simulink model "buffer_tut1"  (Simulink 5.0)
settings: Solver=FixedStepDiscrete  StartTime=0.0  StopTime=10.0  RelTol=1e-3
libraries: dspbuff3 x1, dspxfrm3 x1, dspsrcs4 x1
settings Model: CovMetricSettings=d  Creator=ckamachi  LastModifiedBy=ckamachi  ExtModeTrigMode=oneshot  ExtModeArmWhenConnect=off  LimitDataPoints=off  BlockReductionOpt=off  BooleanDataType=off

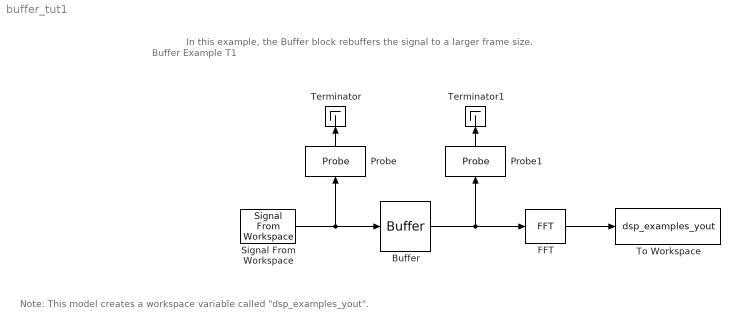
== system buffer_tut1 ==
  note: Buffer Example T1
  note: In this example, the Buffer block rebuffers the signal to a larger frame size.
  note: Note: This model creates a workspace variable called "dsp_examples_yout".
  Buffer : dspbuff3/Buffer  N=16  V=0  ic=0
  FFT : dspxfrm3/FFT  CompMethod=Table lookup  TableOpt=Speed  BitRevOrder=off
  Probe : Probe  Orientation=up  ProbeWidth=off  ProbeComplexSignal=off
  Probe1 : Probe  Orientation=up  ProbeWidth=off  ProbeComplexSignal=off
  Signal From Workspace : dspsrcs4/Signal From Workspace  X=1:1000  Ts=0.125  nsamps=8  OutputAfterFinalValue=Setting to zero
  Terminator : Terminator
      settings: Orientation=up
  Terminator1 : Terminator
      settings: Orientation=up
  To Workspace : ToWorkspace  VariableName=dsp_examples_yout  SampleTime=-1  SaveFormat=Array
  wires:
  FFT/1 -> To Workspace/1
  Signal From Workspace/1 -> Buffer/1, Probe/1
  Buffer/1 -> FFT/1, Probe1/1
  Probe/1 -> Terminator/1
  Probe1/1 -> Terminator1/1
